simulink model "observer"  (R2015b)
settings: Solver=ode23t  StartTime=0.0  StopTime=50  RelTol=1e-3
undefined symbols (not defined in the file): a, A, alpha, D, DaZV_A1, DaZV_A2, DaZV_tau1, DaZV_tau2, delay, N, P, T, tau
libraries: simulink x5, cstblocks x3
settings Model: Creator=dave  LastModifiedBy=dave

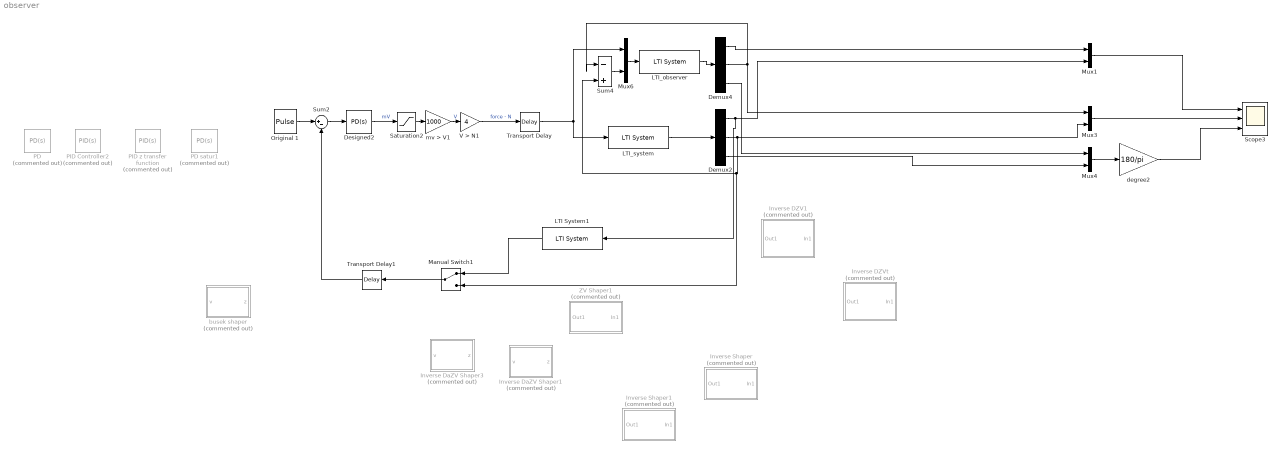
== system observer ==
  Demux2 : Demux  Outputs=3
  Demux4 : Demux  Outputs=3
  Designed2 : simulink/Continuous/PID Controller  Controller=PD  TimeDomain=Continuous-time  SampleTime=-1  IntegratorMethod=Forward Euler  FilterMethod=Forward Euler  Form=Parallel  UseFilter=on  ControllerParametersSource=internal  P=P  I=0.00421956018261364  D=D  N=N  InitialConditionSource=internal  InitialConditionForIntegrator=0  InitialConditionForFilter=0  ExternalReset=none  LimitOutput=off  UpperSaturationLimit=5/1000  LowerSaturationLimit=-5/1000  LinearizeAsGain=on  AntiWindupMode=none  Kb=1  TrackingMode=off  Kt=1  PParamMin=[]  PParamMax=[]  IParamMin=[]  IParamMax=[]  DParamMin=[]  DParamMax=[]  NParamMin=[]  NParamMax=[]  KbParamMin=[]  KbParamMax=[]  KtParamMin=[]  KtParamMax=[]  POutMin=[]  POutMax=[]  IOutMin=[]  IOutMax=[]  DOutMin=[]  DOutMax=[]  NOutMin=[]  NOutMax=[]  KbOutMin=[]  KbOutMax=[]  KtOutMin=[]  KtOutMax=[]  IntegratorOutMin=[]  IntegratorOutMax=[]  FilterOutMin=[]  FilterOutMax=[]  SumOutMin=[]  SumOutMax=[]  SumI1OutMin=[]  SumI1OutMax=[]  SumI2OutMin=[]  SumI2OutMax=[]  SumI3OutMin=[]  SumI3OutMax=[]  SumDOutMin=[]  SumDOutMax=[]  SaturationOutMin=[]  SaturationOutMax=[]  IntegratorContinuousStateAttributes=''  IntegratorStateMustResolveToSignalObject=off  IntegratorRTWStateStorageClass=Auto  FilterContinuousStateAttributes=''  FilterStateMustResolveToSignalObject=off  FilterRTWStateStorageClass=Auto  DifferentiatorICPrevScaledInput=0  DifferentiatorOutMin=[]  DifferentiatorOutMax=[]
  Inverse DZV1 : Subsystem  Commented=on
  Inverse DZVt : Subsystem  Commented=on
  Inverse DaZV Shaper1 : Subsystem  Commented=on
  Inverse DaZV Shaper3 : Subsystem  Commented=on
  Inverse Shaper : Subsystem  Commented=on
  Inverse Shaper1 : Subsystem  Commented=on
  LTI System1 : cstblocks/LTI System  sys=DZV_inv  IC=[]
  LTI_observer : cstblocks/LTI System  sys=observer_ss  IC=[]
  LTI_system : cstblocks/LTI System  sys=system_ss  IC=[]
  Manual Switch1 : ManualSwitch
  Mux{1,3..4,6} (4 alike) : Mux  Inputs=2
  Original 1 : DiscretePulseGenerator  PulseType=Time based  Amplitude=0.15  Period=50  PulseWidth=50
  PD : simulink/Continuous/PID Controller  Commented=on  Controller=PD  TimeDomain=Continuous-time  SampleTime=-1  IntegratorMethod=Forward Euler  FilterMethod=Forward Euler  Form=Parallel  UseFilter=on  ControllerParametersSource=internal  P=0.0394462582002743  I=0.0175856984919557  D=0.00806681081154374  N=12.5569783346429  InitialConditionSource=internal  InitialConditionForIntegrator=0  InitialConditionForFilter=0  ExternalReset=none  LimitOutput=off  UpperSaturationLimit=inf  LowerSaturationLimit=-inf  LinearizeAsGain=on  AntiWindupMode=none  Kb=1  TrackingMode=off  Kt=1  PParamMin=[]  PParamMax=[]  IParamMin=[]  IParamMax=[]  DParamMin=[]  DParamMax=[]  NParamMin=[]  NParamMax=[]  KbParamMin=[]  KbParamMax=[]  KtParamMin=[]  KtParamMax=[]  POutMin=[]  POutMax=[]  IOutMin=[]  IOutMax=[]  DOutMin=[]  DOutMax=[]  NOutMin=[]  NOutMax=[]  KbOutMin=[]  KbOutMax=[]  KtOutMin=[]  KtOutMax=[]  IntegratorOutMin=[]  IntegratorOutMax=[]  FilterOutMin=[]  FilterOutMax=[]  SumOutMin=[]  SumOutMax=[]  SumI1OutMin=[]  SumI1OutMax=[]  SumI2OutMin=[]  SumI2OutMax=[]  SumI3OutMin=[]  SumI3OutMax=[]  SumDOutMin=[]  SumDOutMax=[]  SaturationOutMin=[]  SaturationOutMax=[]  IntegratorContinuousStateAttributes=''  IntegratorStateMustResolveToSignalObject=off  IntegratorRTWStateStorageClass=Auto  FilterContinuousStateAttributes=''  FilterStateMustResolveToSignalObject=off  FilterRTWStateStorageClass=Auto  DifferentiatorICPrevScaledInput=0  DifferentiatorOutMin=[]  DifferentiatorOutMax=[]
  PD satur1 : simulink/Continuous/PID Controller  Commented=on  Controller=PD  TimeDomain=Continuous-time  SampleTime=-1  IntegratorMethod=Forward Euler  FilterMethod=Forward Euler  Form=Parallel  UseFilter=on  ControllerParametersSource=internal  P=0.0609773565396997  I=0.0175856984919557  D=0.00572272711238234  N=12.5569783346429  InitialConditionSource=internal  InitialConditionForIntegrator=0  InitialConditionForFilter=0  ExternalReset=none  LimitOutput=on  UpperSaturationLimit=5/1000  LowerSaturationLimit=-5/1000  LinearizeAsGain=on  AntiWindupMode=none  Kb=1  TrackingMode=off  Kt=1  PParamMin=[]  PParamMax=[]  IParamMin=[]  IParamMax=[]  DParamMin=[]  DParamMax=[]  NParamMin=[]  NParamMax=[]  KbParamMin=[]  KbParamMax=[]  KtParamMin=[]  KtParamMax=[]  POutMin=[]  POutMax=[]  IOutMin=[]  IOutMax=[]  DOutMin=[]  DOutMax=[]  NOutMin=[]  NOutMax=[]  KbOutMin=[]  KbOutMax=[]  KtOutMin=[]  KtOutMax=[]  IntegratorOutMin=[]  IntegratorOutMax=[]  FilterOutMin=[]  FilterOutMax=[]  SumOutMin=[]  SumOutMax=[]  SumI1OutMin=[]  SumI1OutMax=[]  SumI2OutMin=[]  SumI2OutMax=[]  SumI3OutMin=[]  SumI3OutMax=[]  SumDOutMin=[]  SumDOutMax=[]  SaturationOutMin=[]  SaturationOutMax=[]  IntegratorContinuousStateAttributes=''  IntegratorStateMustResolveToSignalObject=off  IntegratorRTWStateStorageClass=Auto  FilterContinuousStateAttributes=''  FilterStateMustResolveToSignalObject=off  FilterRTWStateStorageClass=Auto  DifferentiatorICPrevScaledInput=0  DifferentiatorOutMin=[]  DifferentiatorOutMax=[]
  PID Controller2 : simulink/Continuous/PID Controller  Commented=on  Controller=PID  TimeDomain=Continuous-time  SampleTime=-1  IntegratorMethod=Forward Euler  FilterMethod=Forward Euler  Form=Parallel  UseFilter=on  ControllerParametersSource=internal  P=0.102261702498483  I=0.000537939497443  D=0.00316448395659404  N=1502.67827681922  InitialConditionSource=internal  InitialConditionForIntegrator=0  InitialConditionForFilter=0  ExternalReset=none  LimitOutput=on  UpperSaturationLimit=5/1000  LowerSaturationLimit=-5/1000  LinearizeAsGain=on  AntiWindupMode=none  Kb=1  TrackingMode=off  Kt=1  PParamMin=[]  PParamMax=[]  IParamMin=[]  IParamMax=[]  DParamMin=[]  DParamMax=[]  NParamMin=[]  NParamMax=[]  KbParamMin=[]  KbParamMax=[]  KtParamMin=[]  KtParamMax=[]  POutMin=[]  POutMax=[]  IOutMin=[]  IOutMax=[]  DOutMin=[]  DOutMax=[]  NOutMin=[]  NOutMax=[]  KbOutMin=[]  KbOutMax=[]  KtOutMin=[]  KtOutMax=[]  IntegratorOutMin=[]  IntegratorOutMax=[]  FilterOutMin=[]  FilterOutMax=[]  SumOutMin=[]  SumOutMax=[]  SumI1OutMin=[]  SumI1OutMax=[]  SumI2OutMin=[]  SumI2OutMax=[]  SumI3OutMin=[]  SumI3OutMax=[]  SumDOutMin=[]  SumDOutMax=[]  SaturationOutMin=[]  SaturationOutMax=[]  IntegratorContinuousStateAttributes=''  IntegratorStateMustResolveToSignalObject=off  IntegratorRTWStateStorageClass=Auto  FilterContinuousStateAttributes=''  FilterStateMustResolveToSignalObject=off  FilterRTWStateStorageClass=Auto  DifferentiatorICPrevScaledInput=0  DifferentiatorOutMin=[]  DifferentiatorOutMax=[]
  PID z transfer function : simulink/Continuous/PID Controller  Commented=on  Controller=PID  TimeDomain=Continuous-time  SampleTime=-1  IntegratorMethod=Forward Euler  FilterMethod=Forward Euler  Form=Parallel  UseFilter=on  ControllerParametersSource=internal  P=0.0446452161272428  I=0.00421956018261364  D=0.00573503623999335  N=13.0081121480751  InitialConditionSource=internal  InitialConditionForIntegrator=0  InitialConditionForFilter=0  ExternalReset=none  LimitOutput=on  UpperSaturationLimit=5/1000  LowerSaturationLimit=-5/1000  LinearizeAsGain=on  AntiWindupMode=none  Kb=1  TrackingMode=off  Kt=1  PParamMin=[]  PParamMax=[]  IParamMin=[]  IParamMax=[]  DParamMin=[]  DParamMax=[]  NParamMin=[]  NParamMax=[]  KbParamMin=[]  KbParamMax=[]  KtParamMin=[]  KtParamMax=[]  POutMin=[]  POutMax=[]  IOutMin=[]  IOutMax=[]  DOutMin=[]  DOutMax=[]  NOutMin=[]  NOutMax=[]  KbOutMin=[]  KbOutMax=[]  KtOutMin=[]  KtOutMax=[]  IntegratorOutMin=[]  IntegratorOutMax=[]  FilterOutMin=[]  FilterOutMax=[]  SumOutMin=[]  SumOutMax=[]  SumI1OutMin=[]  SumI1OutMax=[]  SumI2OutMin=[]  SumI2OutMax=[]  SumI3OutMin=[]  SumI3OutMax=[]  SumDOutMin=[]  SumDOutMax=[]  SaturationOutMin=[]  SaturationOutMax=[]  IntegratorContinuousStateAttributes=''  IntegratorStateMustResolveToSignalObject=off  IntegratorRTWStateStorageClass=Auto  FilterContinuousStateAttributes=''  FilterStateMustResolveToSignalObject=off  FilterRTWStateStorageClass=Auto  DifferentiatorICPrevScaledInput=0  DifferentiatorOutMin=[]  DifferentiatorOutMax=[]
  Saturation2 : Saturate  UpperLimit=5/1000  LowerLimit=-5/1000
  Scope3 : Scope  NumInputPorts=3
  Sum2 : Sum  Inputs=|+-
  Sum4 : Sum  Inputs=|-+
  Transport Delay : TransportDelay  DelayTime=delay
  Transport Delay1 : TransportDelay  DelayTime=delay
  V > N1 : Gain  Gain=4
  ZV Shaper1 : Subsystem  Commented=on
  busek shaper : Subsystem  Commented=on
  degree2 : Gain  Gain=180/pi
  mv > V1 : Gain  Gain=1000
  wires:
  Mux4/1 -> degree2/1
  Mux1/1 -> Scope3/1
  Mux3/1 -> Scope3/2
  degree2/1 -> Scope3/3
  LTI_system/1 -> Demux2/1
  mv > V1/1 -> V > N1/1  "V"
  Designed2/1 -> Saturation2/1  "mV"
  Sum2/1 -> Designed2/1
  Original 1/1 -> Sum2/1
  Saturation2/1 -> mv > V1/1
  V > N1/1 -> Transport Delay/1  "force - N"
  LTI_observer/1 -> Demux4/1
  Demux4/1 -> Mux1/1
  Demux4/2 -> Sum4/1, Mux3/1
  Demux4/3 -> Mux4/1
  Mux6/1 -> LTI_observer/1
  Sum4/1 -> Mux6/2
  LTI System1/1 -> Manual Switch1/1
  Demux2/2 -> Mux3/2, Manual Switch1/2, Sum4/2
  Demux2/3 -> Mux4/2
  Manual Switch1/1 -> Transport Delay1/1
  Demux2/1 -> LTI System1/1, Mux1/2
  Transport Delay/1 -> LTI_system/1, Mux6/1
  Transport Delay1/1 -> Sum2/2

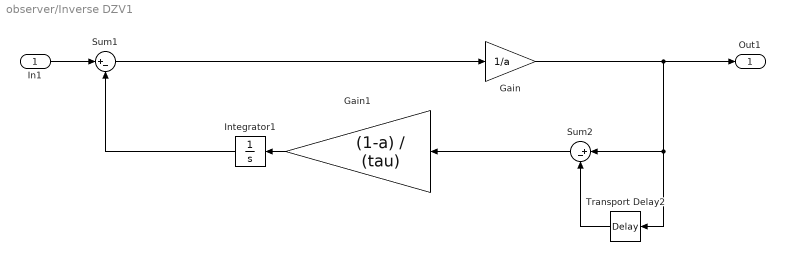
== system observer/Inverse DZV1 ==
  In1 : Inport
  Gain : Gain  Gain=1/a
  Gain1 : Gain  Gain=(1-a) / (tau)
  Integrator1 : Integrator  LimitOutput=on  UpperSaturationLimit=tau  LowerSaturationLimit=0
  Sum1 : Sum  Inputs=|+-
  Sum2 : Sum  Inputs=|+-
  Transport Delay2 : TransportDelay  DelayTime=tau
  Out1 : Outport
  wires:
  Integrator1/1 -> Sum1/2
  Gain/1 -> Out1/1, Transport Delay2/1, Sum2/1
  Transport Delay2/1 -> Sum2/2
  Sum2/1 -> Gain1/1
  In1/1 -> Sum1/1
  Sum1/1 -> Gain/1
  Gain1/1 -> Integrator1/1

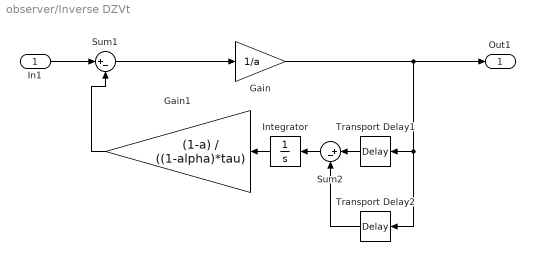
== system observer/Inverse DZVt ==
  In1 : Inport
  Gain : Gain  Gain=1/a
  Gain1 : Gain  Gain=(1-a) / ((1-alpha)*tau)
  Integrator : Integrator  LimitOutput=on  UpperSaturationLimit=tau  LowerSaturationLimit=0
  Sum1 : Sum  Inputs=|+-
  Sum2 : Sum  Inputs=|+-
  Transport Delay1 : TransportDelay  DelayTime=tau*alpha
  Transport Delay2 : TransportDelay  DelayTime=tau
  Out1 : Outport
  wires:
  Transport Delay1/1 -> Sum2/1
  Sum2/1 -> Integrator/1
  Transport Delay2/1 -> Sum2/2
  Integrator/1 -> Gain1/1
  In1/1 -> Sum1/1
  Sum1/1 -> Gain/1
  Gain1/1 -> Sum1/2
  Gain/1 -> Out1/1, Transport Delay1/1, Transport Delay2/1

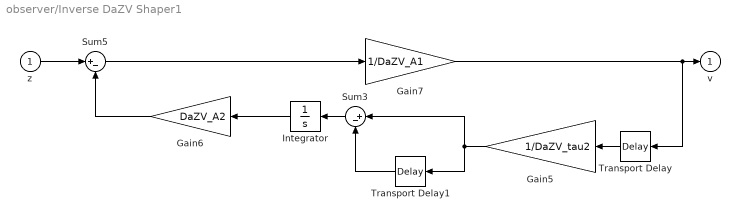
== system observer/Inverse DaZV Shaper1 ==
  z : Inport
  Gain5 : Gain  Gain=1/DaZV_tau2
  Gain6 : Gain  Gain=DaZV_A2
  Gain7 : Gain  Gain=1/DaZV_A1
  Integrator : Integrator
  Sum3 : Sum  Inputs=|+-
  Sum5 : Sum  Inputs=|+-
  Transport Delay : TransportDelay  DelayTime=DaZV_tau1
  Transport Delay1 : TransportDelay  DelayTime=DaZV_tau2
  v : Outport
  wires:
  Sum5/1 -> Gain7/1
  Gain7/1 -> v/1, Transport Delay/1
  Gain6/1 -> Sum5/2
  Integrator/1 -> Gain6/1
  Sum3/1 -> Integrator/1
  Transport Delay1/1 -> Sum3/2
  Gain5/1 -> Transport Delay1/1, Sum3/1
  Transport Delay/1 -> Gain5/1
  z/1 -> Sum5/1

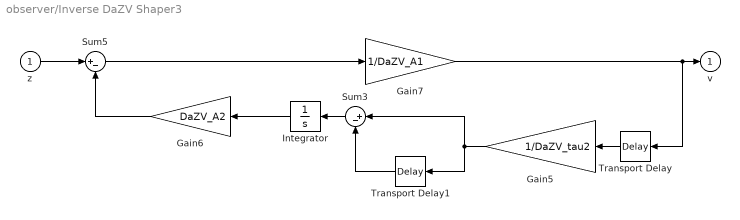
== system observer/Inverse DaZV Shaper3 ==
  z : Inport
  Gain5 : Gain  Gain=1/DaZV_tau2
  Gain6 : Gain  Gain=DaZV_A2
  Gain7 : Gain  Gain=1/DaZV_A1
  Integrator : Integrator
  Sum3 : Sum  Inputs=|+-
  Sum5 : Sum  Inputs=|+-
  Transport Delay : TransportDelay  DelayTime=DaZV_tau1
  Transport Delay1 : TransportDelay  DelayTime=DaZV_tau2
  v : Outport
  wires:
  Sum5/1 -> Gain7/1
  Gain7/1 -> v/1, Transport Delay/1
  Gain6/1 -> Sum5/2
  Integrator/1 -> Gain6/1
  Sum3/1 -> Integrator/1
  Transport Delay1/1 -> Sum3/2
  Gain5/1 -> Transport Delay1/1, Sum3/1
  Transport Delay/1 -> Gain5/1
  z/1 -> Sum5/1

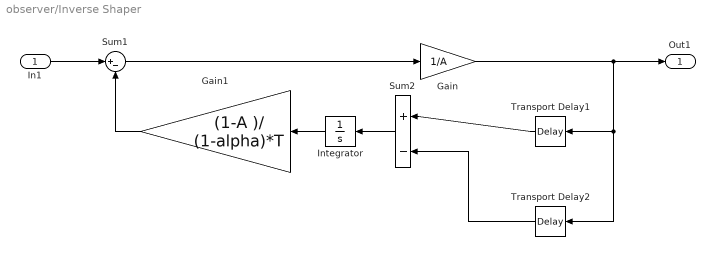
== system observer/Inverse Shaper ==
  In1 : Inport
  Gain : Gain  Gain=1/A
  Gain1 : Gain  Gain=(1-A )/ (1-alpha)*T
  Integrator : Integrator
  Sum1 : Sum  Inputs=|+-
  Sum2 : Sum  Inputs=|+-
  Transport Delay1 : TransportDelay  DelayTime=alpha*tau
  Transport Delay2 : TransportDelay  DelayTime=tau
  Out1 : Outport
  wires:
  Gain/1 -> Transport Delay2/1, Transport Delay1/1, Out1/1
  Gain1/1 -> Sum1/2
  Sum1/1 -> Gain/1
  In1/1 -> Sum1/1
  Integrator/1 -> Gain1/1
  Sum2/1 -> Integrator/1
  Transport Delay1/1 -> Sum2/1
  Transport Delay2/1 -> Sum2/2

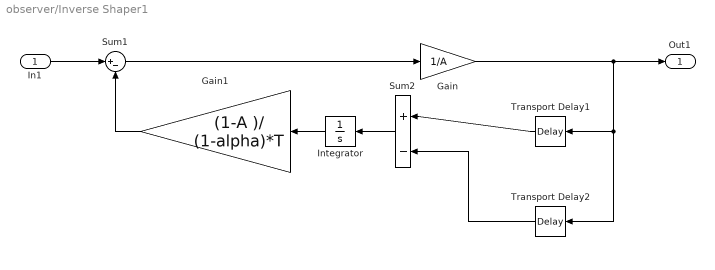
== system observer/Inverse Shaper1 ==
  In1 : Inport
  Gain : Gain  Gain=1/A
  Gain1 : Gain  Gain=(1-A )/ (1-alpha)*T
  Integrator : Integrator
  Sum1 : Sum  Inputs=|+-
  Sum2 : Sum  Inputs=|+-
  Transport Delay1 : TransportDelay  DelayTime=alpha*tau
  Transport Delay2 : TransportDelay  DelayTime=tau
  Out1 : Outport
  wires:
  Transport Delay2/1 -> Sum2/2
  Transport Delay1/1 -> Sum2/1
  Sum2/1 -> Integrator/1
  Integrator/1 -> Gain1/1
  In1/1 -> Sum1/1
  Sum1/1 -> Gain/1
  Gain1/1 -> Sum1/2
  Gain/1 -> Out1/1, Transport Delay1/1, Transport Delay2/1

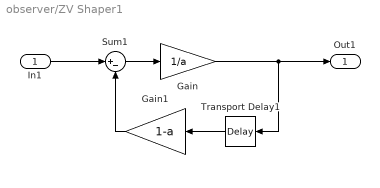
== system observer/ZV Shaper1 ==
  In1 : Inport
  Gain : Gain  Gain=1/a
  Gain1 : Gain  Gain=1-a
  Sum1 : Sum  Inputs=|+-
  Transport Delay1 : TransportDelay  DelayTime=tau
  Out1 : Outport
  wires:
  Transport Delay1/1 -> Gain1/1
  In1/1 -> Sum1/1
  Sum1/1 -> Gain/1
  Gain1/1 -> Sum1/2
  Gain/1 -> Out1/1, Transport Delay1/1

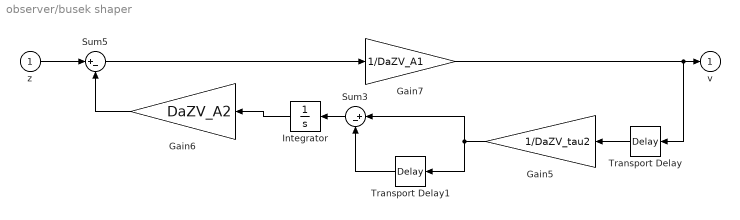
== system observer/busek shaper ==
  z : Inport
  Gain5 : Gain  Gain=1/DaZV_tau2
  Gain6 : Gain  Gain=DaZV_A2
  Gain7 : Gain  Gain=1/DaZV_A1
  Integrator : Integrator
  Sum3 : Sum  Inputs=|+-
  Sum5 : Sum  Inputs=|+-
  Transport Delay : TransportDelay  DelayTime=DaZV_tau1
  Transport Delay1 : TransportDelay  DelayTime=DaZV_tau2
  v : Outport
  wires:
  Sum5/1 -> Gain7/1
  Gain7/1 -> v/1, Transport Delay/1
  Gain6/1 -> Sum5/2
  Integrator/1 -> Gain6/1
  Sum3/1 -> Integrator/1
  Transport Delay1/1 -> Sum3/2
  Gain5/1 -> Transport Delay1/1, Sum3/1
  Transport Delay/1 -> Gain5/1
  z/1 -> Sum5/1
